simulink model "decoder"  (R2015a)
settings: Solver=FixedStepDiscrete  StartTime=0.0  StopTime=300  FixedStep=1  RelTol=1e-3
settings Model: Creator=qiji  LastModifiedBy=qiji
settings OptimizationCC: BlockReduction=off  ConditionallyExecuteInputs=off
settings DebuggingCC: UnderspecifiedInitializationDetection=Classic  MergeDetectMultiDrivingBlocksExec=none  SolverPrmCheckMsg=warning  SingleTaskRateTransMsg=error

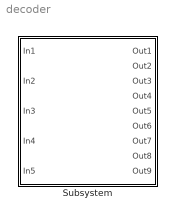
== system decoder ==
  Subsystem : Subsystem

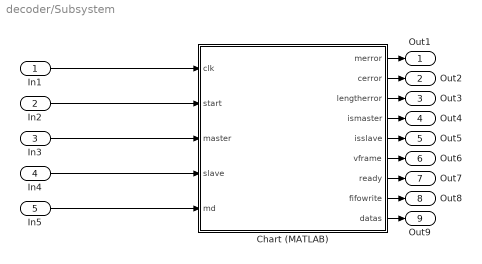
== system decoder/Subsystem ==
  In1 : Inport
  In2 : Inport  Port=2
  In3 : Inport  Port=3
  In4 : Inport  Port=4
  In5 : Inport  Port=5
  Chart (MATLAB) : Stateflow chart  TreatAsAtomicUnit=on
  Out1 : Outport
  Out2 : Outport  Port=2
  Out3 : Outport  Port=3
  Out4 : Outport  Port=4
  Out5 : Outport  Port=5
  Out6 : Outport  Port=6
  Out7 : Outport  Port=7
  Out8 : Outport  Port=8
  Out9 : Outport  Port=9
  wires:
  Chart (MATLAB)/2(cerror) -> Out2/1
  Chart (MATLAB)/5(isslave) -> Out5/1
  Chart (MATLAB)/7(ready) -> Out7/1
  Chart (MATLAB)/8(fifowrite) -> Out8/1
  In3/1 -> Chart (MATLAB)/3(master)
  Chart (MATLAB)/3(lengtherror) -> Out3/1
  In4/1 -> Chart (MATLAB)/4(slave)
  In2/1 -> Chart (MATLAB)/2(start)
  Chart (MATLAB)/9(datas) -> Out9/1
  Chart (MATLAB)/6(vframe) -> Out6/1
  In1/1 -> Chart (MATLAB)/1(clk)
  Chart (MATLAB)/1(merror) -> Out1/1
  Chart (MATLAB)/4(ismaster) -> Out4/1
  In5/1 -> Chart (MATLAB)/5(md)

== stateflow chart decoder/Subsystem/Chart (MATLAB) ==
  settings: executeAtInitialization=1  initializeOutput=1
  state s000Action [function]
    (default) -> (junction 43) : {
        | checkcode=[false; false; false; false;...
        |     false; false; false; false];
        | dataRegisters=[false; false; false; false;...
        |     false; false; false; false;...
        |     false; false; false; false;...
        |     false; false; false; false;];
        | samples = [false; false; false; false];
        | total=[false; false; false];
        | merror=false;
        | cerror=false;
        | ismaster=false;
        | isslave=false;
        | ready=false;
        | fifowrite=false;
        | datas=[false; false; false; false;...
        |     false; false; false; false;...
        |     false; false; false; false;...
        |     false; false; false; false;];
        | cerrorflag=false;
        | cfl=[false; false; false; false; false];
        | overflow=false;
        | lengtherror=false;
        | vframe=false;
        | }
  note: 采样4位以后，开始解码
  state s000
    en:
    masterframe=false;
    slaveframe=false;
    sample8 = uint8(0);
    du:
    s000Action();
    exit:
    s000Action();
  state s001
    s001 -> s001 [order 1] : [clk==1]
        | {
        | sample8=sample8+1;
        | sAction();
        | }
  state s101
    state s01
    state s00
    (junction 86) -> s01 : {
        | dataRegisters(3:16) =...
        |  dataRegisters(1:14);
        | dataRegisters(1:2) = [false; false];
        | frameAction();
        | }
    s00 -> (junction 86) [order 2] : [samples(1)==false &&...
        | samples(2)== true &&...
        | samples(3) == false &&...
        | samples(4) == true]
    s00 -> (junction 87) [order 3] : [samples(1)==false &&...
        | samples(2)== true &&...
        | samples(3) == true &&...
        | samples(4) == false]
    (junction 87) -> s01 : {
        | dataRegisters(3:16) =...
        |  dataRegisters(1:14);
        | dataRegisters(1:2) = [false,true];
        | frameAction();
        | }
    (default) -> s00
    s00 -> (junction 88) [order 5] : [samples(1)==true &&...
        | samples(2)== false &&...
        | samples(3) == false &&...
        | samples(4) == true]
    (junction 88) -> s01 : {
        | dataRegisters(3:16) = ...
        | dataRegisters(1:14);
        | dataRegisters(1:2) =[true,false];
        | frameAction();
        | }
    (junction 89) -> s01 : {
        | dataRegisters(3:16) = ...
        | dataRegisters(0:13);
        | dataRegisters(1:2) =  [true,true];
        | frameAction();
        | }
    s00 -> (junction 89) [order 4] : [samples(1)==true &&...
        | samples(2)== false &&...
        | samples(3) == true &&...
        | samples(4) == false]
  state s100
    s100 -> s100 [order 1] : [clk==1]
        | {
        | sample8 = sample8+1;
        | sAction();
        | }
  state frameAction [function]
    (default) -> (junction 66)
    (junction 66) -> (junction 64) [order 1] : [counter8==7]
    (junction 66) -> (junction 63) [order 2] : {counter8 = counter8+1;}
    (junction 64) -> (junction 65) : {counter8=uint8(0);}
    (junction 65) -> (junction 63)
    (junction 63) -> (junction 71) : {
        | merror=false;
        | cerror=false;
        | ismaster=false;
        | isslave=false;
        | ready=false;
        | lengtherror=false;
        | vframe=false;
        | }
  state s010
    s010 -> s010 [order 1] : [clk==1]
        | {
        | sample8 = sample8+1;
        | sAction();
        | }
  state s011
    s011 -> s011 [order 1] : [clk==1]
        | {
        | sample8 = sample8+1;
        | sAction();
        | }
  state sAction [function]
    (default) -> (junction 58) : {
        | merror=false;
        | cerror=false;
        | ismaster=false;
        | isslave=false;
        | ready=false;
        | fifowrite=false;
        | datas=[false; false; false; false;...
        |     false; false; false; false;...
        |     false; false; false; false;...
        |     false; false; false; false;];
        | lengtherror=false;
        | vframe=false;
        | }
  s00 -> s000 [order 1] : [(samples(1)==false &&...
      | samples(2)== true &&...
      | samples(3) == false &&...
      | samples(4) == true) ||...
      | ...
      | (samples(1)==false &&...
      | samples(2)== true &&...
      | samples(3) == true &&...
      | samples(4) == false) ||...
      | ...
      | (samples(1)==true &&...
      | samples(2)== false &&...
      | samples(3) == false &&...
      | samples(4) == true) ||...
      | ...
      | (samples(1)==true &&...
      | samples(2)== false &&...
      | samples(3) == true &&...
      | samples(4) == false)]
  s000 -> s001 : [start == true]
      | {
      | masterframe=master;
      | slaveframe=slave;
      | sample8=uint8(1);
      | }
  s100 -> s101 [order 1] : [clk==1 && sample8 == 7]
  (default) -> s000
  s001 -> s010 [order 1] : [clk==1 && sample8 == 7]
      | {
      | samples = cat(1, samples(2:4), md);
      | sample8 = uint8(0);
      | sAction();
      | }
  s011 -> s100 [order 1] : [clk==1 && sample8 == 7]
      | {
      | samples = cat(1, samples(2:4), md);
      | sample8 = uint8(0);
      | sAction();
      | }
  s010 -> s011 [order 1] : [clk==1 && sample8==7]
      | {
      | samples = cat(1, samples(2:4), md);
      | sample8 = uint8(0);
      | sAction();
      | }
  data: merror output boolean; cerror output boolean; lengtherror output boolean; ismaster output boolean; isslave output boolean; vframe output boolean; ready output boolean; fifowrite output boolean; datas output boolean size=16; checkcode local boolean size=8; dataRegisters local boolean size=16; masterframe local boolean; slaveframe local boolean; samples local boolean size=4; total local boolean size=3; counter8 local uint8; sample8 local uint8; cerrorflag local boolean; overflow local boolean; cfl local boolean size=5; clk input boolean; start input boolean; master input boolean; slave input boolean; md input boolean
  data checkcode settings: description=存放checkcode
  data dataRegisters settings: description=存放manchester解码后的数据
  data masterframe settings: description=the symbol of master frame
  data slaveframe settings: description=the symbol of slave frame
  data samples settings: description=store 4 bits sample value
  data total settings: description=add 1 per 16 bit
  data counter8 settings: description=the number of data in dataRegisters
  data sample8 settings: description=sample the value per 8 cycle
  data cerrorflag settings: description=标识符：标识校验码错误；‘1’表示有校验码错误，‘0’表示没有检验码错误
  data overflow settings: description=溢出标识位：‘1’表示有溢出，‘0’表示没有溢出
